simulink model "TestStructure"  (R2023b)
settings: Solver=FixedStepDiscrete  StartTime=0.0  StopTime=inf  FixedStep=SampleTime  RelTol=1e-3
InitFcn:
  | SampleTime = 0.001;
  | ButtonValue=0;
  | load("BusConfig.mat");
undefined symbols (not defined in the file): DiscIntNeverNeededParam
libraries: slrealtimeethercatlib x219, dspfdesign x28, dspstat3 x23, simulink x21, slpidlib x10, dspswit3 x8, commfilt2 x2, dspsigops x1
(part 2 of 8)

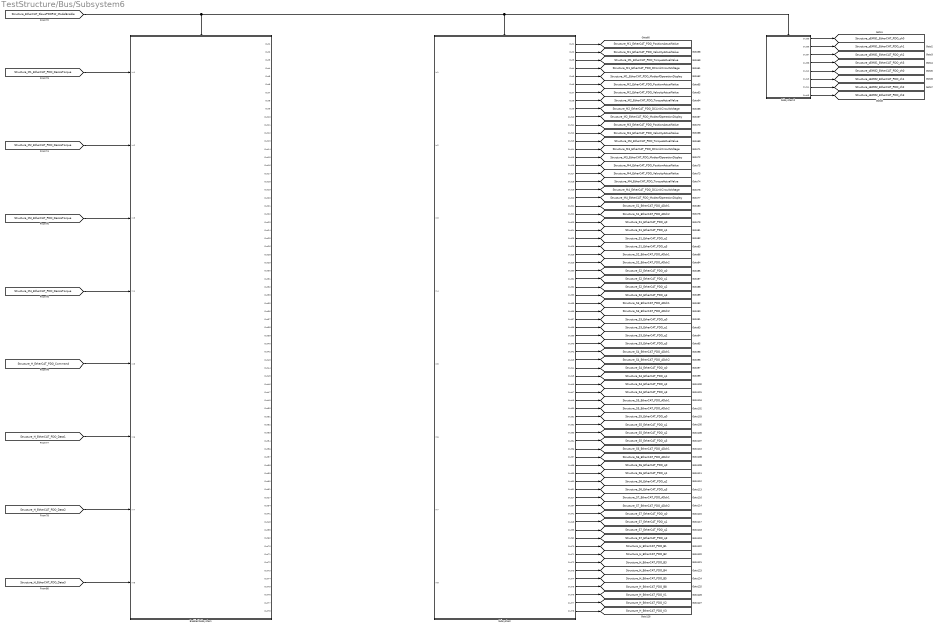
== system TestStructure/Bus/Subsystem6 ==
  Enabled Subsystem : Subsystem  TreatAsAtomicUnit=on
  Subsystem : Subsystem
  Subsystem2 : Subsystem
  tag scope: Structure_H_EtherCAT_PDO_B1=global, Structure_H_EtherCAT_PDO_B2=global, Structure_H_EtherCAT_PDO_B3=global, Structure_H_EtherCAT_PDO_B4=global, Structure_H_EtherCAT_PDO_B5=global, Structure_H_EtherCAT_PDO_B8=global, Structure_H_EtherCAT_PDO_K1=global, Structure_H_EtherCAT_PDO_K2=global, Structure_H_EtherCAT_PDO_K3=global, Structure_M1_EtherCAT_PDO_DCLinkCircuitVoltage=global, Structure_M1_EtherCAT_PDO_ModeofOperationDisplay=global, Structure_M1_EtherCAT_PDO_PositionActualValue=global, Structure_M1_EtherCAT_PDO_TorqueActualValue=global, Structure_M1_EtherCAT_PDO_VelocityActualValue=global, Structure_M2_EtherCAT_PDO_DCLinkCircuitVoltage=global, Structure_M2_EtherCAT_PDO_ModeofOperationDisplay=global, Structure_M2_EtherCAT_PDO_PositionActualValue=global, Structure_M2_EtherCAT_PDO_TorqueActualValue=global, Structure_M2_EtherCAT_PDO_VelocityActualValue=global, Structure_M3_EtherCAT_PDO_DCLinkCircuitVoltage=global, Structure_M3_EtherCAT_PDO_ModeofOperationDisplay=global, Structure_M3_EtherCAT_PDO_PositionActualValue=global, Structure_M3_EtherCAT_PDO_TorqueActualValue=global, Structure_M3_EtherCAT_PDO_VelocityActualValue=global, Structure_M4_EtherCAT_PDO_DCLinkCircuitVoltage=global, Structure_M4_EtherCAT_PDO_ModeofOperationDisplay=global, Structure_M4_EtherCAT_PDO_PositionActualValue=global, Structure_M4_EtherCAT_PDO_TorqueActualValue=global, Structure_M4_EtherCAT_PDO_VelocityActualValue=global, Structure_S1_EtherCAT_PDO_ADch1=global, Structure_S1_EtherCAT_PDO_ADch2=global, Structure_S1_EtherCAT_PDO_q0=global, Structure_S1_EtherCAT_PDO_q1=global, Structure_S1_EtherCAT_PDO_q2=global, Structure_S1_EtherCAT_PDO_q3=global, Structure_S2_EtherCAT_PDO_ADch1=global, Structure_S2_EtherCAT_PDO_ADch2=global, Structure_S2_EtherCAT_PDO_q0=global, Structure_S2_EtherCAT_PDO_q1=global, Structure_S2_EtherCAT_PDO_q2=global, Structure_S2_EtherCAT_PDO_q3=global, Structure_S3_EtherCAT_PDO_ADch1=global, Structure_S3_EtherCAT_PDO_ADch2=global, Structure_S3_EtherCAT_PDO_q0=global, Structure_S3_EtherCAT_PDO_q1=global, Structure_S3_EtherCAT_PDO_q2=global, Structure_S3_EtherCAT_PDO_q3=global, Structure_S4_EtherCAT_PDO_ADch1=global, Structure_S4_EtherCAT_PDO_ADch2=global, Structure_S4_EtherCAT_PDO_q0=global, Structure_S4_EtherCAT_PDO_q1=global, Structure_S4_EtherCAT_PDO_q2=global, Structure_S4_EtherCAT_PDO_q3=global, Structure_S5_EtherCAT_PDO_ADch1=global, Structure_S5_EtherCAT_PDO_ADch2=global, Structure_S5_EtherCAT_PDO_q0=global, Structure_S5_EtherCAT_PDO_q1=global, Structure_S5_EtherCAT_PDO_q2=global, Structure_S5_EtherCAT_PDO_q3=global, Structure_S6_EtherCAT_PDO_ADch1=global, Structure_S6_EtherCAT_PDO_ADch2=global, Structure_S6_EtherCAT_PDO_q0=global, Structure_S6_EtherCAT_PDO_q1=global, Structure_S6_EtherCAT_PDO_q2=global, Structure_S6_EtherCAT_PDO_q3=global, Structure_S7_EtherCAT_PDO_ADch1=global, Structure_S7_EtherCAT_PDO_ADch2=global, Structure_S7_EtherCAT_PDO_q0=global, Structure_S7_EtherCAT_PDO_q1=global, Structure_S7_EtherCAT_PDO_q2=global, Structure_S7_EtherCAT_PDO_q3=global, Structure_sEMG1_EtherCAT_PDO_ch0=global, Structure_sEMG1_EtherCAT_PDO_ch1=global, Structure_sEMG1_EtherCAT_PDO_ch2=global, Structure_sEMG1_EtherCAT_PDO_ch3=global, Structure_sEMG2_EtherCAT_PDO_ch0=global, Structure_sEMG2_EtherCAT_PDO_ch1=global, Structure_sEMG2_EtherCAT_PDO_ch2=global, Structure_sEMG2_EtherCAT_PDO_ch3=global
  wires:
  [Structure_EtherCAT_SlavePDORW_ModelEnable] -> Subsystem2/Enable, Subsystem/Enable, Enabled Subsystem/Enable
  [Structure_M1_EtherCAT_PDO_DesireTorque] -> Enabled Subsystem/1(In1)
  [Structure_M2_EtherCAT_PDO_DesireTorque] -> Enabled Subsystem/2(In2)
  [Structure_M3_EtherCAT_PDO_DesireTorque] -> Enabled Subsystem/3(In3)
  [Structure_M4_EtherCAT_PDO_DesireTorque] -> Enabled Subsystem/4(In4)
  [Structure_H_EtherCAT_PDO_Command] -> Enabled Subsystem/5(In5)
  [Structure_H_EtherCAT_PDO_Data1] -> Enabled Subsystem/6(In6)
  [Structure_H_EtherCAT_PDO_Data2] -> Enabled Subsystem/7(In7)
  [Structure_H_EtherCAT_PDO_Data3] -> Enabled Subsystem/8(In8)
  Subsystem/1(Out1) -> [Structure_M1_EtherCAT_PDO_PositionActualValue]
  Subsystem/2(Out2) -> [Structure_M1_EtherCAT_PDO_VelocityActualValue]
  Subsystem/3(Out3) -> [Structure_M1_EtherCAT_PDO_TorqueActualValue]
  Subsystem/4(Out4) -> [Structure_M1_EtherCAT_PDO_DCLinkCircuitVoltage]
  Subsystem/5(Out5) -> [Structure_M1_EtherCAT_PDO_ModeofOperationDisplay]
  Subsystem/6(Out6) -> [Structure_M2_EtherCAT_PDO_PositionActualValue]
  Subsystem/7(Out7) -> [Structure_M2_EtherCAT_PDO_VelocityActualValue]
  Subsystem/8(Out8) -> [Structure_M2_EtherCAT_PDO_TorqueActualValue]
  Subsystem/9(Out9) -> [Structure_M2_EtherCAT_PDO_DCLinkCircuitVoltage]
  Subsystem/10(Out10) -> [Structure_M2_EtherCAT_PDO_ModeofOperationDisplay]
  Subsystem/11(Out11) -> [Structure_M3_EtherCAT_PDO_PositionActualValue]
  Subsystem/12(Out12) -> [Structure_M3_EtherCAT_PDO_VelocityActualValue]
  Subsystem/13(Out13) -> [Structure_M3_EtherCAT_PDO_TorqueActualValue]
  Subsystem/14(Out14) -> [Structure_M3_EtherCAT_PDO_DCLinkCircuitVoltage]
  Subsystem/15(Out15) -> [Structure_M3_EtherCAT_PDO_ModeofOperationDisplay]
  Subsystem/16(Out16) -> [Structure_M4_EtherCAT_PDO_PositionActualValue]
  Subsystem/17(Out17) -> [Structure_M4_EtherCAT_PDO_VelocityActualValue]
  Subsystem/18(Out18) -> [Structure_M4_EtherCAT_PDO_TorqueActualValue]
  Subsystem/19(Out19) -> [Structure_M4_EtherCAT_PDO_DCLinkCircuitVoltage]
  Subsystem/20(Out20) -> [Structure_M4_EtherCAT_PDO_ModeofOperationDisplay]
  Subsystem/21(Out21) -> [Structure_S1_EtherCAT_PDO_ADch1]
  Subsystem/22(Out22) -> [Structure_S1_EtherCAT_PDO_ADch2]
  Subsystem/23(Out23) -> [Structure_S1_EtherCAT_PDO_q0]
  Subsystem/24(Out24) -> [Structure_S1_EtherCAT_PDO_q1]
  Subsystem/25(Out25) -> [Structure_S1_EtherCAT_PDO_q2]
  Subsystem/26(Out26) -> [Structure_S1_EtherCAT_PDO_q3]
  Subsystem/27(Out28) -> [Structure_S2_EtherCAT_PDO_ADch1]
  Subsystem/28(Out29) -> [Structure_S2_EtherCAT_PDO_ADch2]
  Subsystem/29(Out30) -> [Structure_S2_EtherCAT_PDO_q0]
  Subsystem/30(Out31) -> [Structure_S2_EtherCAT_PDO_q1]
  Subsystem/31(Out32) -> [Structure_S2_EtherCAT_PDO_q2]
  Subsystem/32(Out33) -> [Structure_S2_EtherCAT_PDO_q3]
  Subsystem/33(Out35) -> [Structure_S3_EtherCAT_PDO_ADch1]
  Subsystem/34(Out36) -> [Structure_S3_EtherCAT_PDO_ADch2]
  Subsystem/35(Out37) -> [Structure_S3_EtherCAT_PDO_q0]
  Subsystem/36(Out38) -> [Structure_S3_EtherCAT_PDO_q1]
  Subsystem/37(Out39) -> [Structure_S3_EtherCAT_PDO_q2]
  Subsystem/38(Out40) -> [Structure_S3_EtherCAT_PDO_q3]
  Subsystem/39(Out42) -> [Structure_S4_EtherCAT_PDO_ADch1]
  Subsystem/40(Out43) -> [Structure_S4_EtherCAT_PDO_ADch2]
  Subsystem/41(Out44) -> [Structure_S4_EtherCAT_PDO_q0]
  Subsystem/42(Out45) -> [Structure_S4_EtherCAT_PDO_q1]
  Subsystem/43(Out46) -> [Structure_S4_EtherCAT_PDO_q2]
  Subsystem/44(Out47) -> [Structure_S4_EtherCAT_PDO_q3]
  Subsystem/45(Out49) -> [Structure_S5_EtherCAT_PDO_ADch1]
  Subsystem/46(Out50) -> [Structure_S5_EtherCAT_PDO_ADch2]
  Subsystem/47(Out51) -> [Structure_S5_EtherCAT_PDO_q0]
  Subsystem/48(Out52) -> [Structure_S5_EtherCAT_PDO_q1]
  Subsystem/49(Out53) -> [Structure_S5_EtherCAT_PDO_q2]
  Subsystem/50(Out54) -> [Structure_S5_EtherCAT_PDO_q3]
  Subsystem/51(Out56) -> [Structure_S6_EtherCAT_PDO_ADch1]
  Subsystem/52(Out57) -> [Structure_S6_EtherCAT_PDO_ADch2]
  Subsystem/53(Out58) -> [Structure_S6_EtherCAT_PDO_q0]
  Subsystem/54(Out59) -> [Structure_S6_EtherCAT_PDO_q1]
  Subsystem/55(Out60) -> [Structure_S6_EtherCAT_PDO_q2]
  Subsystem/56(Out61) -> [Structure_S6_EtherCAT_PDO_q3]
  Subsystem/57(Out27) -> [Structure_S7_EtherCAT_PDO_ADch1]
  Subsystem/58(Out34) -> [Structure_S7_EtherCAT_PDO_ADch2]
  Subsystem/59(Out41) -> [Structure_S7_EtherCAT_PDO_q0]
  Subsystem/60(Out48) -> [Structure_S7_EtherCAT_PDO_q1]
  Subsystem/61(Out55) -> [Structure_S7_EtherCAT_PDO_q2]
  Subsystem/62(Out62) -> [Structure_S7_EtherCAT_PDO_q3]
  Subsystem/63(Out70) -> [Structure_H_EtherCAT_PDO_B1]
  Subsystem/64(Out71) -> [Structure_H_EtherCAT_PDO_B2]
  Subsystem/65(Out72) -> [Structure_H_EtherCAT_PDO_B3]
  Subsystem/66(Out73) -> [Structure_H_EtherCAT_PDO_B4]
  Subsystem/67(Out74) -> [Structure_H_EtherCAT_PDO_B5]
  Subsystem/68(Out75) -> [Structure_H_EtherCAT_PDO_B8]
  Subsystem/69(Out76) -> [Structure_H_EtherCAT_PDO_K1]
  Subsystem/70(Out77) -> [Structure_H_EtherCAT_PDO_K2]
  Subsystem/71(Out78) -> [Structure_H_EtherCAT_PDO_K3]
  Subsystem2/1(Out35) -> [Structure_sEMG1_EtherCAT_PDO_ch0]
  Subsystem2/2(Out36) -> [Structure_sEMG1_EtherCAT_PDO_ch1]
  Subsystem2/3(Out37) -> [Structure_sEMG1_EtherCAT_PDO_ch2]
  Subsystem2/4(Out38) -> [Structure_sEMG1_EtherCAT_PDO_ch3]
  Subsystem2/5(Out42) -> [Structure_sEMG2_EtherCAT_PDO_ch0]
  Subsystem2/6(Out43) -> [Structure_sEMG2_EtherCAT_PDO_ch1]
  Subsystem2/7(Out44) -> [Structure_sEMG2_EtherCAT_PDO_ch2]
  Subsystem2/8(Out45) -> [Structure_sEMG2_EtherCAT_PDO_ch3]

== system TestStructure/Bus/Subsystem7 ==
  Enabled Subsystem : Subsystem  Commented=on  TreatAsAtomicUnit=on
  Enabled Subsystem1 : Subsystem  Commented=on  TreatAsAtomicUnit=on
  Enabled Subsystem2 : Subsystem  Commented=on  TreatAsAtomicUnit=on
  Enabled Subsystem3 : Subsystem  Commented=on  TreatAsAtomicUnit=on
  Enabled Subsystem4 : Subsystem  Commented=on  TreatAsAtomicUnit=on
  Enabled Subsystem5 : Subsystem  Commented=on  TreatAsAtomicUnit=on
  Enabled Subsystem6 : Subsystem  Commented=on  TreatAsAtomicUnit=on
  Enabled Subsystem7 : Subsystem  Commented=on  TreatAsAtomicUnit=on
  tag scope: Structure_M4_EtherCAT_GetDeviceState_State=global, Structure_M4_EtherCAT_Init_PDO_PositionActualValue=global, Structure_M4_EtherCAT_PDO_StatusWord=global, Structure_M4_EtherCAT_SDO_6060_Error=global, Structure_M4_EtherCAT_SDO_6060_Status=global, Structure_M4_EtherCAT_SDO_6075_Data=global, Structure_M4_EtherCAT_SDO_6075_Error=global, Structure_M4_EtherCAT_SDO_6075_Status=global, Structure_M4_EtherCAT_SDO_6080_Error=global, Structure_M4_EtherCAT_SDO_6080_Status=global, Structure_M4_EtherCAT_SetDeviceState1_Error=global, Structure_M4_EtherCAT_SetDeviceState1_PrevState=global, Structure_M4_EtherCAT_SetDeviceState_Error=global, Structure_M4_EtherCAT_SetDeviceState_PrevState=global
  wires:
  [Structure_M4_EtherCAT_SetDeviceState_ModelEnable] -> Enabled Subsystem/Enable
  [Structure_M4_EtherCAT_SDO_6075_ModelEnable] -> Enabled Subsystem1/Enable
  [Structure_M4_EtherCAT_SDO_6080_ModelEnable] -> Enabled Subsystem2/Enable
  [Structure_M4_EtherCAT_SDO_6060_ModelEnable] -> Enabled Subsystem3/Enable
  [Structure_M4_EtherCAT_SetDeviceState1_ModelEnable] -> Enabled Subsystem4/Enable
  [Structure_M4_EtherCAT_InitReadPos_ModelEnable] -> Enabled Subsystem7/Enable
  [Structure_M4_EtherCAT_PDO_6040_ModelEnable] -> Enabled Subsystem6/Enable
  [Structure_M4_EtherCAT_GetDeviceState_ModelEnable] -> Enabled Subsystem5/Enable
  [Structure_M4_EtherCAT_SetDeviceState_NewState] -> Enabled Subsystem/1(In1)
  [Structure_M4_EtherCAT_SetDeviceState_Enable] -> Enabled Subsystem/2(In2)
  Enabled Subsystem/1(Out1) -> [Structure_M4_EtherCAT_SetDeviceState_PrevState]
  Enabled Subsystem/2(Out2) -> [Structure_M4_EtherCAT_SetDeviceState_Error]
  [Structure_M4_EtherCAT_SDO_6075_Enable] -> Enabled Subsystem1/1(In3)
  Enabled Subsystem1/1(Out3) -> [Structure_M4_EtherCAT_SDO_6075_Data]
  Enabled Subsystem1/2(Out4) -> [Structure_M4_EtherCAT_SDO_6075_Status]
  Enabled Subsystem1/3(Out5) -> [Structure_M4_EtherCAT_SDO_6075_Error]
  [Structure_M4_EtherCAT_SDO_6080_Enable] -> Enabled Subsystem2/2(In5)
  [Structure_M4_EtherCAT_SDO_6080_Data] -> Enabled Subsystem2/1(In4)
  Enabled Subsystem2/2(Out7) -> [Structure_M4_EtherCAT_SDO_6080_Error]
  Enabled Subsystem2/1(Out6) -> [Structure_M4_EtherCAT_SDO_6080_Status]
  [Structure_M4_EtherCAT_SDO_6060_Data] -> Enabled Subsystem3/1(In6)
  [Structure_M4_EtherCAT_SDO_6060_Enable] -> Enabled Subsystem3/2(In7)
  Enabled Subsystem3/1(Out8) -> [Structure_M4_EtherCAT_SDO_6060_Status]
  Enabled Subsystem3/2(Out9) -> [Structure_M4_EtherCAT_SDO_6060_Error]
  [Structure_M4_EtherCAT_SetDeviceState1_NewState] -> Enabled Subsystem4/1(In8)
  [Structure_M4_EtherCAT_SetDeviceState1_Enable] -> Enabled Subsystem4/2(In9)
  Enabled Subsystem4/1(Out10) -> [Structure_M4_EtherCAT_SetDeviceState1_PrevState]
  Enabled Subsystem4/2(Out11) -> [Structure_M4_EtherCAT_SetDeviceState1_Error]
  Enabled Subsystem5/1(Out12) -> [Structure_M4_EtherCAT_GetDeviceState_State]
  [Structure_M4_EtherCAT_PDO_ControlWord] -> Enabled Subsystem6/1(In10)
  Enabled Subsystem6/1(Out13) -> [Structure_M4_EtherCAT_PDO_StatusWord]
  Enabled Subsystem7/1(Out1) -> [Structure_M4_EtherCAT_Init_PDO_PositionActualValue]

== system TestStructure/InterForceControlTask/AO ==
  q : Inport
  sEMGMuxIn : Inport  Port=2
  PhaseBias : Inport  Port=3
  Whichfoot : Inport  Port=4
  ColdStartEventClock : DigitalClock  SampleTime=0.001
  ColdStartEventGate : MATLAB Function  TreatAsAtomicUnit=on
  Constant : Constant
  Constant1 : Constant
  Demux : Demux  Outputs=3
  Filter : Subsystem
  Gain : Gain  Gain=0.01
  MATLAB Function : MATLAB Function  TreatAsAtomicUnit=on
  Memory : Memory
  PhaseCorrection : Subsystem
      settings: PortSchema="{\"entries\":[{\"content\":{\"sides\":[{\"content\":{\"connectorIds\":[\"In1\"]},\"type\":\"ConnectorPlacement.EquallySpacedRectSide\",\"uuid\":\"a940d053-290e-486f-ae2d-d4bfa32c46e0\"},{\"content\":{\"connectorIds\":[\"Out1\",\"Out2\"],\"side\":\"RIGHT\"},\"type\":\"ConnectorPlacement.EquallySpacedRectSide\",\"uuid\":\"a83f9ff7-c6c8-4eeb-9804-d4a4971b2c0c\"},{\"content\":{\"side\":\"TOP\"},\"type\":\"ConnectorPlacement.EquallySpacedRectSide\",\"uuid\":\"31fb4f87-600a-4f18-9d17-ff98d57e3413\"},{\"content\":{\"connectorIds\":[\"In2\"],\"side\":\"BOTTOM\"},\"type\":\"ConnectorPlacement.EquallySpacedRectSide\",\"uuid\":\"7c261045-8ba1-4ca6-a6a7-b959d0e37f01\"}]},\"type\":\"ConnectorPlacement.EquallySpacedConnector\",\"uuid\":\"19432f00-0669-4bb6-9210-56124374c33b\"}],\"packageUris\":[\"http://schema.mathworks.com/mf0/Connector/R2020b\"],\"version\":\"1.0\"}"
  Select : Subsystem
  Subsystem1 : Subsystem
  Switch : Switch  Criteria=u2 > Threshold  SaturateOnIntegerOverflow=off  InputSameDT=off
  TBaseDefault : Constant  Value=2.2
  FeetLoad : Outport
  x : Outport  Port=2
  Omega : Outport  Port=3
  Phi : Outport  Port=4
  Phase0Event : Outport  Port=5
  wires:
  Memory/1 -> MATLAB Function/1(phi)
  Select/3(PhaseEn) -> Subsystem1/Enable
  Constant1/1 -> Select/1(P)
  PhaseCorrection/1(Omega) -> Omega/1
  Gain/1 -> Select/3(q), Subsystem1/1(q)
  Select/1(Phi_Out) -> Phi/1
  MATLAB Function/1(y) -> Select/2(Phi)
  PhaseCorrection/2(Phi_Corrected) -> Memory/1
  PhaseBias/1 -> MATLAB Function/2(deltaphi)
  Filter/1(Out) -> Gain/1
  Subsystem1/2(Peak) -> PhaseCorrection/1(Peaks)
  sEMGMuxIn/1 -> Subsystem1/2(sEMGMuxIn)
  Whichfoot/1 -> Subsystem1/3(Whichfoot)
  Subsystem1/3(FeetLoad) -> FeetLoad/1
  q/1 -> Demux/1
  Demux/2 -> Switch/2  "which"
  Demux/1 -> Switch/1  "left"
  Demux/3 -> Switch/3  "right"
  Switch/1 -> Filter/1(In)
  TBaseDefault/1 -> PhaseCorrection/2(T_base_default), ColdStartEventGate/3(T_base_default)
  Select/2(Phase0Event) -> Phase0Event/1, ColdStartEventGate/1(event_in)
  ColdStartEventClock/1 -> ColdStartEventGate/2(t_now)
  ColdStartEventGate/1(event_out) -> ?

== system TestStructure/InterForceControlTask/AO1 ==
  q : Inport
  PhaseBias : Inport  Port=2
  Bias : Bias  Bias=-30  SaturateOnIntegerOverflow=off
  Constant : Constant
  Constant1 : Constant
  Filter : Subsystem
  Gain : Gain  Gain=0.01
  MATLAB Function : MATLAB Function  TreatAsAtomicUnit=on
  Memory : Memory
  PhaseCorrection : Subsystem
  Select : Subsystem
  Subsystem : Subsystem  Commented=on
  Subsystem1 : Subsystem
  x : Outport
  Omega : Outport  Port=2
  Phi : Outport  Port=3
  Phase0Event : Outport  Port=4
  wires:
  Memory/1 -> MATLAB Function/1(phi)
  Subsystem1/2(Peak) -> PhaseCorrection/1(Peaks)
  Select/3(PhaseEn) -> Subsystem1/Enable
  Constant1/1 -> Select/1(P)
  PhaseCorrection/1(Omega) -> Omega/1
  Gain/1 -> Subsystem1/1(q), Select/3(q)
  Select/2(Phase0Event) -> Phase0Event/1
  Select/1(Phi_Out) -> Phi/1
  MATLAB Function/1(y) -> Select/2(Phi)
  PhaseCorrection/2(Phi_Corrected) -> Memory/1
  PhaseBias/1 -> MATLAB Function/2(deltaphi)
  Bias/1 -> ?
  Filter/1(Out) -> Gain/1, Bias/1
  q/1 -> Filter/1(In)

== system TestStructure/InterForceControlTask/AO2 ==
  q : Inport
  PhaseBias : Inport  Port=2
  Bias : Bias  Bias=-30  SaturateOnIntegerOverflow=off
  Filter : Subsystem
  Gain : Gain  Gain=0.01
  MATLAB Function : MATLAB Function  TreatAsAtomicUnit=on
  PhaseCorrection : Subsystem
      settings: PortSchema="{\"entries\":[{\"content\":{\"sides\":[{\"content\":{\"connectorIds\":[\"In1\"]},\"type\":\"ConnectorPlacement.EquallySpacedRectSide\",\"uuid\":\"29c766a6-008c-4672-8933-7f2b92d9002e\"},{\"content\":{\"connectorIds\":[\"Out1\"],\"side\":\"RIGHT\"},\"type\":\"ConnectorPlacement.EquallySpacedRectSide\",\"uuid\":\"ebf4015b-900d-44c2-b090-12eb3718c736\"},{\"content\":{\"connectorIds\":[\"In2\",\"In3\",\"In4\"],\"side\":\"TOP\"},\"type\":\"ConnectorPlacement.EquallySpacedRectSide\",\"uuid\":\"76801015-3401-4c32-9066-c2a5e8571b2e\"},{\"content\":{\"side\":\"BOTTOM\"},\"type\":\"ConnectorPlacement.EquallySpacedRectSide\",\"uuid\":\"4a70095e-69af-4392-aa02-795a2e72b843\"}]},\"type\":\"ConnectorPlacement.EquallySpacedConnector\",\"uuid\":\"005c6ef6-da38-46d8-8867-20bf9861f3d8\"}],\"packageUris\":[\"http://schema.mathworks.com/mf0/Connector/R2020b\"],\"version\":\"1.0\"}"
  Select : Subsystem
  Subsystem : Subsystem
  Subsystem1 : Subsystem
  x : Outport
  Omega : Outport  Port=2
  Phi : Outport  Port=3
  Phase0Event : Outport  Port=4
  wires:
  Select/2(Phase0Event) -> Phase0Event/1
  Select/1(Phi_Out) -> Phi/1
  MATLAB Function/1(y) -> Select/2(Phi)
  Subsystem/4(P) -> Select/1(P)
  PhaseCorrection/1(Phi_Corrected) -> MATLAB Function/1(phi)
  Subsystem/3(Phi) -> PhaseCorrection/2(Phi_GP)
  Subsystem/2(Omega) -> PhaseCorrection/3(Omega), Omega/1
  PhaseBias/1 -> MATLAB Function/2(deltaphi)
  Subsystem1/1(f) -> Subsystem/2(f)
  Bias/1 -> ?
  Gain/1 -> Subsystem1/1(q), Select/3(q), Subsystem/1(q)
  Filter/1(Out) -> Gain/1, Bias/1
  Subsystem1/2(Peak) -> PhaseCorrection/1(Peaks)
  q/1 -> Filter/1(In)
  Subsystem/1(x) -> x/1

== system TestStructure/InterForceControlTask/AO3 ==
  q : Inport
  PhaseBias : Inport  Port=2
  Bias : Bias  Bias=-30  SaturateOnIntegerOverflow=off
  Constant : Constant
  Constant1 : Constant
  Filter : Subsystem
  Gain : Gain  Gain=0.01
  MATLAB Function : MATLAB Function  TreatAsAtomicUnit=on
  PhaseCorrection : Subsystem
  Select : Subsystem
  Subsystem : Subsystem  Commented=on
  Subsystem1 : Subsystem
  x : Outport
  Omega : Outport  Port=2
  Phi : Outport  Port=3
  Phase0Event : Outport  Port=4
  wires:
  Constant1/1 -> Select/1(P)
  PhaseCorrection/1(Omega) -> Omega/1
  Constant/1 -> Select/3(q)
  Select/2(Phase0Event) -> Phase0Event/1
  Select/1(Phi_Out) -> Phi/1
  MATLAB Function/1(y) -> Select/2(Phi)
  PhaseCorrection/2(Phi_Corrected) -> MATLAB Function/1(phi)
  PhaseBias/1 -> MATLAB Function/2(deltaphi)
  Bias/1 -> ?
  Gain/1 -> Subsystem1/1(q)
  Filter/1(Out) -> Gain/1, Bias/1
  Subsystem1/2(Peak) -> PhaseCorrection/1(Peaks)
  q/1 -> Filter/1(In)

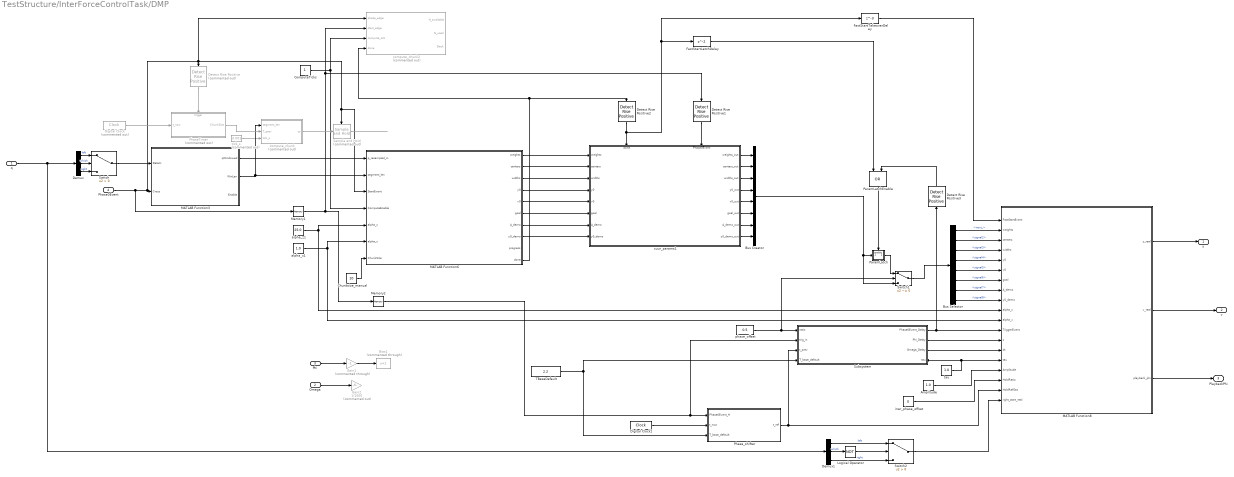
== system TestStructure/InterForceControlTask/DMP ==
  q : Inport
  Omega : Inport  Port=2
  Phi : Inport  Port=3
  Phase0Event : Inport  Port=4
  Amplitude : Constant  Value=1.0
  Bias1 : Bias  Commented=through  Bias=1  SaturateOnIntegerOverflow=off
  Bus Creator : BusCreator  Inputs=8
  Bus Selector : BusSelector  OutputSignals=next_,signal2,signal3,signal4,signal5,signal6,signal7,signal8
  Chunksize_manual : Constant  Value=10
  ComputeTicks : Constant
  Demux : Demux  Outputs=3
  Demux1 : Demux  Outputs=3
  Detect Rise Positive : simulink/Logic and Bit Operations/Detect Rise Positive  Commented=on  vinit=0  OutDataTypeStr=boolean
  Detect Rise Positive1 : simulink/Logic and Bit Operations/Detect Rise Positive  vinit=0  OutDataTypeStr=boolean
  Detect Rise Positive2 : simulink/Logic and Bit Operations/Detect Rise Positive  vinit=0  OutDataTypeStr=boolean
  Detect Rise Positive3 : simulink/Logic and Bit Operations/Detect Rise Positive  vinit=0  OutDataTypeStr=boolean
  Digital Clock : DigitalClock  Commented=on  SampleTime=0.001
  Digital Clock1 : DigitalClock  SampleTime=0.001
  FastStartLatchDelay : Delay  InitialCondition=0
  FastStartTakeoverDelay : Delay  DelayLength=3  InitialCondition=0
  Gain1 : Gain  Commented=through  Gain=-1
  Gain2 : Gain  Commented=on  Gain=1/1000
  Logical Operator : Logic  Operator=NOT  AllPortsSameDT=off  OutDataTypeStr=boolean
  MATLAB Function3 : MATLAB Function  TreatAsAtomicUnit=on
  MATLAB Function6 : MATLAB Function  TreatAsAtomicUnit=on
  MATLAB Function8 : MATLAB Function  TreatAsAtomicUnit=on
  Memory1 : Memory
  Memory2 : Memory
  ParamLatch : Subsystem  TreatAsAtomicUnit=on
  ParamLatchEnable : Logic  Operator=OR  AllPortsSameDT=off  OutDataTypeStr=boolean
  PhaseTimer : Subsystem  Commented=on  TreatAsAtomicUnit=on
  Phase_shifter : MATLAB Function  TreatAsAtomicUnit=on
  Sample and Hold : dspsigops/Sample and Hold  Commented=on  trig=Rising edge  initCond=0  latchinput=off
  Subsystem : Subsystem
      settings: PortSchema="{\"entries\":[{\"content\":{\"sides\":[{\"content\":{\"connectorIds\":[\"In1\",\"In2\",\"In3\",\"In4\"]},\"type\":\"ConnectorPlacement.EquallySpacedRectSide\",\"uuid\":\"1070cfcb-3ec5-4141-8951-8c3ef1706a2a\"},{\"content\":{\"connectorIds\":[\"Out1\",\"Out2\",\"Out3\",\"In5\"],\"side\":\"RIGHT\"},\"type\":\"ConnectorPlacement.EquallySpacedRectSide\",\"uuid\":\"bed4e625-42d0-4ea4-b6d1-bbd729333a1c\"},{\"content\":{\"side\":\"TOP\"},\"type\":\"ConnectorPlacement.EquallySpacedRectSide\",\"uuid\":\"c279c2b1-2727-4963-bce9-c67f4ee7a970\"}]},\"type\":\"ConnectorPlacement.EquallySpacedConnector\",\"uuid\":\"94e6fa59-a73d-4cda-bb27-ca572fd247c8\"}],\"packageUris\":[\"http://schema.mathworks.com/mf0/Connector/R2020b\"],\"version\":\"1.0\"}"
  Switch : Switch  Criteria=u2 > Threshold  SaturateOnIntegerOverflow=off  InputSameDT=off
  Switch1 : Switch  Criteria=u2 ~= 0  SaturateOnIntegerOverflow=off  InputSameDT=off
  Switch2 : Switch  Criteria=u2 > Threshold  SaturateOnIntegerOverflow=off  InputSameDT=off
  TBaseDefault : Constant  Value=2.2
  alpha_x1 : Constant  Value=1.0
  alpha_z1 : Constant  Value=25.0
  compute_chunk : MATLAB Function  Commented=on  TreatAsAtomicUnit=on
  compute_chunk2 : MATLAB Function  Commented=on  TreatAsAtomicUnit=on
  cuur_params1 : Subsystem  TreatAsAtomicUnit=on
      settings: PortSchema="{\"entries\":[{\"content\":{\"sides\":[{\"content\":{\"connectorIds\":[\"In1\",\"In2\",\"In3\",\"In4\",\"In5\",\"In6\",\"In7\",\"In8\"]},\"type\":\"ConnectorPlacement.EquallySpacedRectSide\",\"uuid\":\"3d372f5a-e7b4-49e3-b2c9-9176d5cbfa33\"},{\"content\":{\"connectorIds\":[\"Out1\",\"Out2\",\"Out3\",\"Out4\",\"Out5\",\"Out6\",\"Out7\",\"Out8\"],\"side\":\"RIGHT\"},\"type\":\"ConnectorPlacement.EquallySpacedRectSide\",\"uuid\":\"ee9298d3-2ae2-4770-892a-2c75b17955ec\"},{\"content\":{\"connectorIds\":[\"In9\",\"In10\"],\"side\":\"TOP\"},\"type\":\"ConnectorPlacement.EquallySpacedRectSide\",\"uuid\":\"d0638e77-81ba-40cc-8800-354c93838fef\"}]},\"type\":\"ConnectorPlacement.EquallySpacedConnector\",\"uuid\":\"50317f07-3edb-4206-bc08-c56b750c0251\"}],\"packageUris\":[\"http://schema.mathworks.com/mf0/Connector/R2020b\"],\"version\":\"1.0\"}"
  iner_phase_offset : Constant  Value=0
  phase_offset : Constant  Value=0.5
  tau : Constant  Value=1.0
  tick_s : Constant  Commented=on  Value=0.001
  y : Outport
  v : Outport  Port=2
  PlaybackPhi : Outport  Port=3
  wires:
  MATLAB Function8/2(v_real) -> v/1
  Subsystem/2(Phi_Delay) -> MATLAB Function8/13(s)
  Subsystem/1(Phase0Event_Delay) -> MATLAB Function8/12(TriggerEvent), Detect Rise Positive3/1
  Subsystem/3(Omega_Delay) -> MATLAB Function8/14(dt)
  Bus Selector/8 -> MATLAB Function8/9(y0_demo)  "<signal8>"
  Bus Selector/7 -> MATLAB Function8/8(A_demo)  "<signal7>"
  Bus Selector/6 -> MATLAB Function8/7(goal)  "<signal6>"
  Bus Selector/5 -> MATLAB Function8/6(v0)  "<signal5>"
  Bus Selector/4 -> MATLAB Function8/5(y0)  "<signal4>"
  Bus Selector/3 -> MATLAB Function8/4(widths)  "<signal3>"
  Bus Selector/2 -> MATLAB Function8/3(centers)  "<signal2>"
  Bus Selector/1 -> MATLAB Function8/2(weights)  "<next_>"
  Switch1/1 -> Bus Selector/1
  ParamLatch/1(Out1) -> Switch1/1
  phase_offset/1 -> Switch1/2, Subsystem/1(ratio)
  Detect Rise Positive3/1 -> ParamLatchEnable/2
  Bus Creator/1 -> Switch1/3, ParamLatch/1(In1)
  MATLAB Function8/1(y_real) -> y/1
  cuur_params1/8(y0_demo_out) -> Bus Creator/8
  cuur_params1/7(A_demo_out) -> Bus Creator/7
  cuur_params1/6(goal_out) -> Bus Creator/6
  cuur_params1/5(v0_out) -> Bus Creator/5
  cuur_params1/4(y0_out) -> Bus Creator/4
  cuur_params1/3(widths_out) -> Bus Creator/3
  cuur_params1/2(centers_out) -> Bus Creator/2
  cuur_params1/1(weights_out) -> Bus Creator/1
  iner_phase_offset/1 -> MATLAB Function8/17(HoldRatio)
  Phase_shifter/1(t_ref) -> MATLAB Function8/18(HoldRefSec), Subsystem/3(t_prev)
  Digital Clock1/1 -> Phase_shifter/2(t_now)
  Chunksize_manual/1 -> MATLAB Function6/7(ChunkSize)
  ComputeTicks/1 -> MATLAB Function6/4(ComputeEnable), compute_chunk2/3(compute_tick)
  q/1 -> Demux1/1, Demux/1
  MATLAB Function6/2(centers) -> cuur_params1/2(centers)
  Gain1/1 -> Bias1/1
  MATLAB Function6/6(goal) -> cuur_params1/6(goal)
  Phase0Event/1 -> Memory1/1, MATLAB Function3/2(Cross), Detect Rise Positive/1, MATLAB Function6/3(StartEvent), Sample and Hold/Trigger, compute_chunk2/1(phase_edge)
  MATLAB Function3/1(qWindowed) -> MATLAB Function6/1(p_resampled_in)
  alpha_x1/1 -> MATLAB Function6/6(alpha_x), MATLAB Function8/11(alpha_x)
  Digital Clock/1 -> PhaseTimer/1(t_now)
  tick_s/1 -> compute_chunk/3(tick_s)
  alpha_z1/1 -> MATLAB Function6/5(alpha_z), MATLAB Function8/10(alpha_z)
  Omega/1 -> Gain2/1
  MATLAB Function6/7(A_demo) -> cuur_params1/7(A_demo)
  MATLAB Function6/5(v0) -> cuur_params1/5(v0)
  MATLAB Function3/2(WinLen) -> MATLAB Function6/2(segment_len), compute_chunk/1(segment_len)
  Memory1/1 -> Memory2/1, compute_chunk2/2(start_edge), Detect Rise Positive1/1
  tau/1 -> MATLAB Function8/15(tau), Subsystem/5(tau)
  Amplitude/1 -> MATLAB Function8/16(Amplitude)
  Sample and Hold/1 -> ?
  Detect Rise Positive/1 -> PhaseTimer/Trigger
  MATLAB Function6/8(y0_demo) -> cuur_params1/8(y0_demo)
  Phi/1 -> Gain1/1
  Detect Rise Positive2/1 -> FastStartLatchDelay/1, FastStartTakeoverDelay/1, cuur_params1/9(done)
  MATLAB Function6/4(y0) -> cuur_params1/4(y0)
  MATLAB Function6/1(weights) -> cuur_params1/1(weights)
  MATLAB Function6/10(done) -> Detect Rise Positive2/1, compute_chunk2/4(done)
  Detect Rise Positive1/1 -> cuur_params1/10(Phase0Event)
  compute_chunk/1(cs) -> Sample and Hold/1
  PhaseTimer/1(ChunkSize) -> compute_chunk/2(T_prev)
  Memory2/1 -> Phase_shifter/1(Phase0Event_H), Subsystem/2(trig_in)
  MATLAB Function6/3(widths) -> cuur_params1/3(widths)
  Switch2/1 -> MATLAB Function8/19(right_start_real)
  MATLAB Function8/3(playback_phi) -> PlaybackPhi/1
  TBaseDefault/1 -> Phase_shifter/3(T_base_default), Subsystem/4(T_base_default)
  FastStartLatchDelay/1 -> ParamLatchEnable/1
  ParamLatchEnable/1 -> ParamLatch/Enable
  FastStartTakeoverDelay/1 -> MATLAB Function8/1(FastStartEvent)
  Demux/3 -> Switch/3  "right"
  Demux/2 -> Switch/2  "which"
  Demux/1 -> Switch/1  "left"
  Switch/1 -> MATLAB Function3/1(DataIn)
  Demux1/3 -> Switch2/3  "right"
  Demux1/2 -> Logical Operator/1  "which"
  Demux1/1 -> Switch2/1  "left"
  Logical Operator/1 -> Switch2/2

== system TestStructure/InterForceControlTask/FootSwitch ==
  <LeftHipMotorActuralPosition> : Inport
  <LeftHipMotorActuralVelocity> : Inport  Port=2
  <RightHipMotorActuralPosition> : Inport  Port=3
  <RightHipMotorActuralVelocity> : Inport  Port=4
  <FootSelect> : Inport  Port=5
  Mux : Mux  Inputs=3
  Switch1 : Switch  Criteria=u2 > Threshold  SaturateOnIntegerOverflow=off  InputSameDT=off
  Switch2 : Switch  Criteria=u2 > Threshold  SaturateOnIntegerOverflow=off  InputSameDT=off
  ActuralPosition : Outport
  ActuralVelocity : Outport  Port=2
  q : Outport  Port=3
  wires:
  <LeftHipMotorActuralPosition>/1 -> Mux/1, Switch1/3
  <LeftHipMotorActuralVelocity>/1 -> Switch2/3
  <RightHipMotorActuralPosition>/1 -> Switch1/1, Mux/3
  <RightHipMotorActuralVelocity>/1 -> Switch2/1
  <FootSelect>/1 -> Mux/2, Switch2/2, Switch1/2
  Mux/1 -> q/1
  Switch1/1 -> ActuralPosition/1
  Switch2/1 -> ActuralVelocity/1

== system TestStructure/InterForceControlTask/TorqueController ==
  q_meas : Inport
  dq_meas : Inport  Port=2
  q_ref : Inport  Port=3
  dq_ref : Inport  Port=4
  Abs : Abs  SaturateOnIntegerOverflow=off
  Activity gate : Merge
  Activity_Enable : Constant
  Clock : Clock
  Filter1 : Subsystem
  Gain : Gain  Gain=0.01
  Gain3 : Gain  Gain=0.4
  If : If  NumInputs=2  IfExpression=(u1 >= u2)
  If Action Subsystem1 : Subsystem  TreatAsAtomicUnit=on
  If Action Subsystem_activity_on : Subsystem  TreatAsAtomicUnit=on
  MATLAB Function1 : MATLAB Function  TreatAsAtomicUnit=on
  MATLAB Function2 : MATLAB Function  TreatAsAtomicUnit=on
  MATLAB Function3 : MATLAB Function  TreatAsAtomicUnit=on
  MO_ActivityMovent : Sum
  MO_ActivtyThreadhold : Constant  Value=0.1
  MO_AutoDisable? : ManualSwitch  CurrentSetting=0
  MO_Kd : Gain  Gain=0.002
  MO_Kp : Gain  Gain=0.15
  Moving Average1 : dspstat3/Moving Average  Method=Sliding window  ForgettingFactorPort=off  SpecifyWindowLength=on  WindowLength=2000  OverlapLength=1999  AllowArbitraryInputLength=off  ForgettingFactor=0.9  SimulateUsing=Code generation
  Subsystem2 : Subsystem
  Sum_e : Sum  Inputs=|++
  Sum_e_dq : Sum  Inputs=|-+
  Sum_e_q : Sum  Inputs=|-+
  TorqueManager : Subsystem
  tau_e : Outport
  wires:
  dq_meas/1 -> Sum_e_dq/1
  q_ref/1 -> Filter1/1(In), Sum_e_q/2
  dq_ref/1 -> Sum_e_dq/2
  Sum_e_q/1 -> MO_Kp/1
  Sum_e_dq/1 -> MO_Kd/1
  MO_Kp/1 -> Sum_e/1
  MO_Kd/1 -> Sum_e/2
  Filter1/1(Out) -> Gain/1
  q_meas/1 -> Sum_e_q/1
  Sum_e/1 -> TorqueManager/3(target_torque)
  Subsystem2/1(Peak) -> TorqueManager/2(valid_peak), MATLAB Function2/1(valid_peak), MATLAB Function1/1(raw_peak)  "MO_DMPPhase0Event"
  Clock/1 -> MATLAB Function1/2(t)
  Gain/1 -> MATLAB Function3/1(u), Subsystem2/1(q)
  Gain3/1 -> MO_ActivityMovent/1
  Abs/1 -> Gain3/1, Moving Average1/1
  Moving Average1/1 -> MO_ActivityMovent/2
  If Action Subsystem1/1(activity_gain) -> Activity gate/1  "1"
  MATLAB Function3/1(y) -> Abs/1
  MO_ActivityMovent/1 -> If/1
  If/1 -> If Action Subsystem1/Action
  MO_ActivtyThreadhold/1 -> If/2
  If/2 -> If Action Subsystem_activity_on/Action
  TorqueManager/1(actual_torque) -> tau_e/1
  If Action Subsystem_activity_on/1(activity_gain) -> Activity gate/2  "0"
  Activity gate/1 -> MO_AutoDisable?/1
  TorqueManager/2(current_gain) -> ?  "MO_currentgain"
  MATLAB Function2/1(total_steps) -> ?  "MO_DMPStepCunter"
  Activity_Enable/1 -> MO_AutoDisable?/2
  MO_AutoDisable?/1 -> TorqueManager/1(activity_enable)

== system TestStructure/InterForceControlTask/TorqueController2 ==
  dq_meas : Inport
  q_meas : Inport  Port=2
  q_ref : Inport  Port=3
  dq_ref : Inport  Port=4
  Clock : Clock
  Filter : Subsystem
  Gain : Gain  Gain=0.01
  Gain_Kd : Gain  Gain=0.005
  Gain_Kp : Gain  Gain=0.3
  MATLAB Function : MATLAB Function  TreatAsAtomicUnit=on
  MATLAB Function1 : MATLAB Function  TreatAsAtomicUnit=on
  MATLAB Function2 : MATLAB Function  TreatAsAtomicUnit=on
  Sum_e : Sum  Inputs=|++
  Sum_e_dq : Sum  Inputs=|-+
  Sum_e_q : Sum  Inputs=|-+
  ZeroCrossFinder_Right : Subsystem
  tau_e : Outport
  wires:
  Clock/1 -> MATLAB Function1/2(t), MATLAB Function/3(t)
  MATLAB Function1/1(valid_peak) -> MATLAB Function/1(valid_peak), MATLAB Function2/1(valid_peak)  "valid_peak_right"
  ZeroCrossFinder_Right/1(peak_right) -> MATLAB Function1/1(raw_peak)  "peak_right"
  MATLAB Function/1(actual_torque) -> tau_e/1
  Gain/1 -> ZeroCrossFinder_Right/1(U)
  q_meas/1 -> Sum_e_q/1
  Filter/1(Out) -> Gain/1
  Sum_e/1 -> MATLAB Function/2(target_torque)
  Gain_Kd/1 -> Sum_e/2
  Gain_Kp/1 -> Sum_e/1
  Sum_e_dq/1 -> Gain_Kd/1
  Sum_e_q/1 -> Gain_Kp/1
  dq_ref/1 -> Sum_e_dq/2
  q_ref/1 -> Sum_e_q/2, Filter/1(q)
  dq_meas/1 -> Sum_e_dq/1

== system TestStructure/InterForceControlTask/Torque_Guard ==
  FeetLoad : Inport
  WhichFoot : Inport  Port=2
  tau_e : Inport  Port=3
  <LeftHipMotorActuralPosition> : Inport  Port=4
  <RightHipMotorActuralPosition> : Inport  Port=5
  "?AllTimeDefault" : ManualSwitch
  ContactRelay : Relay  OnSwitchValue=2.0  OffSwitchValue=1.25
  ContactRelay1 : Relay  OnSwitchValue=2.0  OffSwitchValue=1.25
  Demux : Demux  Outputs=2
  Demux1 : Demux  Outputs=2
  LeftLowPass : DiscreteTransferFcn  Numerator=0.05  Denominator=[1 -0.95]  SampleTime=0.001
  LeftLowPass1 : DiscreteTransferFcn  Numerator=0.05  Denominator=[1 -0.95]  SampleTime=0.001
  LimitProtect : Subsystem
      settings: PortSchema="{\"entries\":[{\"content\":{\"sides\":[{\"content\":{\"connectorIds\":[\"In1\",\"In2\",\"In3\"]},\"type\":\"ConnectorPlacement.EquallySpacedRectSide\",\"uuid\":\"37de08c4-f478-48e2-abb8-0aa49397069a\"},{\"content\":{\"connectorIds\":[\"Out1\",\"Out2\"],\"side\":\"RIGHT\"},\"type\":\"ConnectorPlacement.EquallySpacedRectSide\",\"uuid\":\"c7301fee-e42f-4254-87ba-788286fb640b\"},{\"content\":{\"connectorIds\":[\"In4\",\"In5\"],\"side\":\"TOP\"},\"type\":\"ConnectorPlacement.EquallySpacedRectSide\",\"uuid\":\"b96d884e-d525-4025-9411-9b9f9b32393f\"}]},\"type\":\"ConnectorPlacement.EquallySpacedConnector\",\"uuid\":\"b1e8dc5e-81c3-4a24-8e6d-921b13202a7f\"}],\"packageUris\":[\"http://schema.mathworks.com/mf0/Connector/R2020b\"],\"version\":\"1.0\"}"
  Logical Operator : Logic  Operator=NOT  AllPortsSameDT=off  OutDataTypeStr=boolean
  MO_ConsistantTau : Constant  Value=0
  MO_HealthLegdefault : Constant  Value=4.5
  MinimumTauGate : Subsystem
      settings: PortSchema="{\"entries\":[{\"content\":{\"sides\":[{\"content\":{\"connectorIds\":[\"In1\",\"In2\"]},\"type\":\"ConnectorPlacement.EquallySpacedRectSide\",\"uuid\":\"4d89c13b-f800-4481-b2e6-5754ccd4480d\"},{\"content\":{\"connectorIds\":[\"Out1\"],\"side\":\"RIGHT\"},\"type\":\"ConnectorPlacement.EquallySpacedRectSide\",\"uuid\":\"4c64cb92-33d7-49cd-aa82-02535cb98185\"},{\"content\":{\"side\":\"TOP\"},\"type\":\"ConnectorPlacement.EquallySpacedRectSide\",\"uuid\":\"dafdc7d9-c373-415f-80c5-51ad8948e064\"},{\"content\":{\"connectorIds\":[\"In3\"],\"side\":\"BOTTOM\"},\"type\":\"ConnectorPlacement.EquallySpacedRectSide\",\"uuid\":\"81b2cf25-e4b6-4f36-873c-2716d25d74ab\"}]},\"type\":\"ConnectorPlacement.EquallySpacedConnector\",\"uuid\":\"833ddaaa-290b-4880-823a-aa34ea5ccf1d\"}],\"packageUris\":[\"http://schema.mathworks.com/mf0/Connector/R2020b\"],\"version\":\"1.0\"}"
  SwingTauRelease : Subsystem
      settings: PortSchema="{\"entries\":[{\"content\":{\"sides\":[{\"content\":{\"connectorIds\":[\"In1\",\"In2\"]},\"type\":\"ConnectorPlacement.EquallySpacedRectSide\",\"uuid\":\"4d89c13b-f800-4481-b2e6-5754ccd4480d\"},{\"content\":{\"connectorIds\":[\"Out1\"],\"side\":\"RIGHT\"},\"type\":\"ConnectorPlacement.EquallySpacedRectSide\",\"uuid\":\"4c64cb92-33d7-49cd-aa82-02535cb98185\"},{\"content\":{\"connectorIds\":[\"In3\"],\"side\":\"TOP\"},\"type\":\"ConnectorPlacement.EquallySpacedRectSide\",\"uuid\":\"dafdc7d9-c373-415f-80c5-51ad8948e064\"},{\"content\":{\"side\":\"BOTTOM\"},\"type\":\"ConnectorPlacement.EquallySpacedRectSide\",\"uuid\":\"81b2cf25-e4b6-4f36-873c-2716d25d74ab\"}]},\"type\":\"ConnectorPlacement.EquallySpacedConnector\",\"uuid\":\"833ddaaa-290b-4880-823a-aa34ea5ccf1d\"}],\"packageUris\":[\"http://schema.mathworks.com/mf0/Connector/R2020b\"],\"version\":\"1.0\"}"
  Switch{,1..3} (4 alike) : Switch  Criteria=u2 > Threshold  SaturateOnIntegerOverflow=off  InputSameDT=off
  Right : Outport
  Left : Outport  Port=2
  wires:
  tau_e/1 -> MinimumTauGate/1(tau_e)
  Switch/1 -> LimitProtect/1(LeftHipMotorTorque)
  MO_HealthLegdefault/1 -> MinimumTauGate/2(In2), "?AllTimeDefault"/2, SwingTauRelease/2(In2)
  Switch1/1 -> LimitProtect/2(RightHipMotorTorque)
  LimitProtect/1(LeftHipMotorTorque_safe) -> Left/1
  LimitProtect/2(RightHipMotorTorque_safe) -> Right/1
  <LeftHipMotorActuralPosition>/1 -> LimitProtect/4(<LeftHipMotorActuralPosition>)
  <RightHipMotorActuralPosition>/1 -> LimitProtect/5(<RightHipMotorActuralPosition>)
  MinimumTauGate/1(Out1) -> Switch/3, Switch1/1
  LeftLowPass/1 -> ContactRelay/1
  FeetLoad/1 -> Demux/1, Demux1/1
  Demux/1 -> Switch2/1
  Demux/2 -> Switch2/3
  Logical Operator/1 -> Switch2/2
  Switch2/1 -> LeftLowPass/1
  ContactRelay/1 -> MinimumTauGate/3(In3)  "isAffectedStanding"
  WhichFoot/1 -> Switch1/2, LimitProtect/3(<WhichFoot>), Logical Operator/1, Switch/2, Switch3/2
  Demux1/1 -> Switch3/1
  Demux1/2 -> Switch3/3
  Switch3/1 -> LeftLowPass1/1
  LeftLowPass1/1 -> ContactRelay1/1
  ContactRelay1/1 -> SwingTauRelease/3(In3)  "isHealthyStanding"
  MO_ConsistantTau/1 -> SwingTauRelease/1(tau_e)
  "?AllTimeDefault"/1 -> Switch1/3, Switch/1
  SwingTauRelease/1(Out1) -> "?AllTimeDefault"/1

== system TestStructure/Robot/MotorPositonInit1 ==
  P : Inport
  BusOut : Inport  Port=2  OutDataTypeStr=Bus: SensingBusNew
  Enable : EnablePort
  Bus Creator : BusCreator  Inputs=4  OutDataTypeStr=Bus: ControlBusNew  NonVirtualBus=on
  Bus Selector : BusSelector  OutputSignals=LeftShoulderMotorActuralPosition,LeftShoulderMotorActuralVelocity
  Bus Selector1 : BusSelector  OutputSignals=RightShoulderMotorActuralPosition,RightShoulderMotorActuralVelocity
  Bus Selector2 : BusSelector  OutputSignals=LeftHipMotorActuralPosition,LeftHipMotorActuralVelocity
  Bus Selector3 : BusSelector  OutputSignals=RightHipMotorActuralPosition,RightHipMotorActuralVelocity
  Constant{,2..3,6} (4 alike) : Constant  Value=0
  Constant1 : Constant  OutDataTypeStr=double
  Constant4 : Constant  Value=0  OutDataTypeStr=double
  Constant5 : Constant
  Demux : Demux
  Discrete-Time Integrator : DiscreteIntegrator  SampleTime=-1  ICPrevOutput=DiscIntNeverNeededParam  ICPrevScaledInput=DiscIntNeverNeededParam
  Display5 : Display
  If Action Subsystem5 : Subsystem  TreatAsAtomicUnit=on
  If Action Subsystem6 : Subsystem  TreatAsAtomicUnit=on
  If2 : If  IfExpression=(u1 > 3.6)
  MATLAB Function1 : MATLAB Function  TreatAsAtomicUnit=on
  MATLAB Function2 : MATLAB Function  TreatAsAtomicUnit=on
  MATLAB Function3 : MATLAB Function  TreatAsAtomicUnit=on
  MATLAB Function4 : MATLAB Function  TreatAsAtomicUnit=on
  Merge1 : Merge
  Subsystem : Subsystem  Commented=on
  Subsystem1 : Subsystem
  Subsystem2 : Subsystem
  Subsystem3 : Subsystem
  Subsystem4 : Subsystem
  TaskFinished : Outport
  i_d : Outport  Port=2  OutDataTypeStr=Bus: ControlBusNew
  wires:
  Constant5/1 -> Discrete-Time Integrator/1
  If2/1 -> If Action Subsystem5/Action
  If2/2 -> If Action Subsystem6/Action
  If Action Subsystem6/1(Out1) -> Merge1/2
  Constant4/1 -> If Action Subsystem6/1(In1)
  Constant1/1 -> If Action Subsystem5/1(In1)
  If Action Subsystem5/1(Out1) -> Merge1/1
  Merge1/1 -> TaskFinished/1
  Bus Selector/2 -> Subsystem4/3(MotorVel)  "<LeftShoulderMotorActuralVelocity>"
  Bus Selector1/1 -> Subsystem1/2(MotorPos)  "<RightShoulderMotorActuralPosition>"
  Bus Selector1/2 -> Subsystem1/3(MotorVel)  "<RightShoulderMotorActuralVelocity>"
  MATLAB Function1/1(y) -> Subsystem1/1(MotorDesirePos)
  Constant/1 -> Bus Creator/1  "LeftShoulderMotorTorque"
  Subsystem3/1(MotorTorque) -> Bus Creator/4  "RightHipMotorTorque"
  Subsystem2/1(MotorTorque) -> Bus Creator/3  "LeftHipMotorTorque"
  Constant2/1 -> Bus Creator/2  "RightShoulderMotorTorque"
  Bus Creator/1 -> i_d/1
  BusOut/1 -> Bus Selector3/1, Bus Selector2/1, Bus Selector1/1, Bus Selector/1
  Bus Selector/1 -> Subsystem4/2(MotorPos)  "<LeftShoulderMotorActuralPosition>"
  Discrete-Time Integrator/1 -> MATLAB Function4/2(t), MATLAB Function3/2(t), MATLAB Function1/2(t), MATLAB Function2/2(t), If2/1, Display5/1
  Demux/1 -> MATLAB Function2/1(P)
  Demux/2 -> MATLAB Function1/1(P)
  MATLAB Function2/1(y) -> Subsystem4/1(MotorDesirePos)
  Demux/4 -> MATLAB Function4/1(P)
  Demux/3 -> MATLAB Function3/1(P)
  P/1 -> Demux/1
  Bus Selector2/1 -> Subsystem2/2(MotorPos)  "<LeftHipMotorActuralPosition>"
  Bus Selector2/2 -> Subsystem2/3(MotorVel)  "<LeftHipMotorActuralVelocity>"
  Bus Selector3/1 -> Subsystem3/2(MotorPos)  "<RightHipMotorActuralPosition>"
  Bus Selector3/2 -> Subsystem3/3(MotorVel)  "<RightHipMotorActuralVelocity>"
  MATLAB Function3/1(y) -> Subsystem2/1(MotorDesirePos)
  MATLAB Function4/1(y) -> Subsystem3/1(MotorDesirePos)

== system TestStructure/Bus/Subsystem/Enabled Subsystem ==
  In1 : Inport
  In2 : Inport  Port=2
  Enable : EnablePort
  Set Device State : slrealtimeethercatlib/Set SubDevice State  device_id=0  subdevice_name=Drive 3 (Elmo Drive )  sample_time=-1  subdevice_addr=1003  selected_subdevice=Term 1 (EK1100)  subdevice_found=1
  Out1 : Outport
  Out2 : Outport  Port=2
  wires:
  In1/1 -> Set Device State/1
  Set Device State/2 -> Out2/1
  In2/1 -> Set Device State/2
  Set Device State/1 -> Out1/1

== system TestStructure/Bus/Subsystem/Enabled Subsystem1 ==
  In3 : Inport
  Enable : EnablePort
  EtherCAT Async SDO Upload : slrealtimeethercatlib/EtherCAT Async SDO Upload  index=0x6075  subIndex=0  sig_type=uint32  sig_dim=1  device_id=0  subdevice_name=Drive 3 (Elmo Drive )  sample_time=-1  subdevice_addr=1003  selected_subdevice=Term 1 (EK1100)  timeout=3000  subdevice_found=1  complete=0
  Out3 : Outport
  Out4 : Outport  Port=2
  Out5 : Outport  Port=3
  wires:
  EtherCAT Async SDO Upload/3 -> Out5/1
  In3/1 -> EtherCAT Async SDO Upload/1
  EtherCAT Async SDO Upload/2 -> Out4/1
  EtherCAT Async SDO Upload/1 -> Out3/1

== system TestStructure/Bus/Subsystem/Enabled Subsystem2 ==
  In4 : Inport
  In5 : Inport  Port=2
  Enable : EnablePort
  EtherCAT Async SDO Download : slrealtimeethercatlib/EtherCAT Async SDO Download  index=0x6080  subIndex=0  sig_type=int32  sig_dim=1  device_id=0  subdevice_name=Drive 3 (Elmo Drive )  sample_time=-1  subdevice_addr=1003  selected_subdevice=Term 1 (EK1100)  timeout=3000  subdevice_found=1  complete=0
  Out6 : Outport
  Out7 : Outport  Port=2
  wires:
  EtherCAT Async SDO Download/2 -> Out7/1
  In4/1 -> EtherCAT Async SDO Download/1
  In5/1 -> EtherCAT Async SDO Download/2
  EtherCAT Async SDO Download/1 -> Out6/1

== system TestStructure/Bus/Subsystem/Enabled Subsystem3 ==
  In6 : Inport
  In7 : Inport  Port=2
  Enable : EnablePort
  EtherCAT Async SDO Download1 : slrealtimeethercatlib/EtherCAT Async SDO Download  index=0x6060  subIndex=0  sig_type=int8  sig_dim=1  device_id=0  subdevice_name=Drive 3 (Elmo Drive )  sample_time=-1  subdevice_addr=1003  selected_subdevice=Term 1 (EK1100)  timeout=2000  subdevice_found=1  complete=0
  Out8 : Outport
  Out9 : Outport  Port=2
  wires:
  In6/1 -> EtherCAT Async SDO Download1/1
  EtherCAT Async SDO Download1/1 -> Out8/1
  In7/1 -> EtherCAT Async SDO Download1/2
  EtherCAT Async SDO Download1/2 -> Out9/1

== system TestStructure/Bus/Subsystem/Enabled Subsystem4 ==
  In8 : Inport
  In9 : Inport  Port=2
  Enable : EnablePort
  Set Device State1 : slrealtimeethercatlib/Set SubDevice State  device_id=0  subdevice_name=Drive 3 (Elmo Drive )  sample_time=-1  subdevice_addr=1003  selected_subdevice=Term 1 (EK1100)  subdevice_found=1
  Out10 : Outport
  Out11 : Outport  Port=2
  wires:
  Set Device State1/1 -> Out10/1
  In8/1 -> Set Device State1/1
  In9/1 -> Set Device State1/2
  Set Device State1/2 -> Out11/1

== system TestStructure/Bus/Subsystem/Enabled Subsystem5 ==
  Enable : EnablePort
  Get Device State : slrealtimeethercatlib/Get SubDevice State  device_id=0  subdevice_name=Drive 3 (Elmo Drive )  sample_time=0.001  subdevice_addr=1003  selected_subdevice=Term 1 (EK1100)  timeout=500  subdevice_found=1
  Out12 : Outport
  wires:
  Get Device State/1 -> Out12/1

== system TestStructure/Bus/Subsystem/Enabled Subsystem6 ==
  In10 : Inport
  Enable : EnablePort
  EtherCAT PDO Receive1 : slrealtimeethercatlib/EtherCAT PDO Receive  Priority=2  sig_name=Drive 3 (Elmo Drive ).Inputs.Status word  sig_offset=1480  sig_type=uint16  type_size=16  sig_dim=1  device_id=0  sample_time=0.001000
  EtherCAT PDO Transmit1 : slrealtimeethercatlib/EtherCAT PDO Transmit  Priority=3  sig_name=Drive 3 (Elmo Drive ).Outputs.Control word  sig_offset=1448  sig_type=uint16  type_size=16  sig_dim=1  device_id=0  sample_time=0.001000
  Out13 : Outport
  wires:
  EtherCAT PDO Receive1/1 -> Out13/1
  In10/1 -> EtherCAT PDO Transmit1/1

== system TestStructure/Bus/Subsystem/Enabled Subsystem7 ==
  Enable : EnablePort
  EtherCAT PDO Receive2 : slrealtimeethercatlib/EtherCAT PDO Receive  Priority=2  sig_name=Drive 3 (Elmo Drive ).Inputs.Position actual value  sig_offset=1432  sig_type=int32  type_size=32  sig_dim=1  device_id=0  sample_time=0.001000
  Out1 : Outport
  wires:
  EtherCAT PDO Receive2/1 -> Out1/1

== system TestStructure/Bus/Subsystem4/Enabled Subsystem ==
  In1 : Inport
  In2 : Inport  Port=2
  Enable : EnablePort
  Set Device State : slrealtimeethercatlib/Set SubDevice State  device_id=0  subdevice_name=Drive 6 (Elmo Drive )  sample_time=-1  subdevice_addr=1006  selected_subdevice=Term 1 (EK1100)  subdevice_found=1
  Out1 : Outport
  Out2 : Outport  Port=2
  wires:
  In1/1 -> Set Device State/1
  Set Device State/2 -> Out2/1
  In2/1 -> Set Device State/2
  Set Device State/1 -> Out1/1

== system TestStructure/Bus/Subsystem4/Enabled Subsystem1 ==
  In3 : Inport
  Enable : EnablePort
  EtherCAT Async SDO Upload : slrealtimeethercatlib/EtherCAT Async SDO Upload  index=0x6075  subIndex=0  sig_type=uint32  sig_dim=1  device_id=0  subdevice_name=Drive 6 (Elmo Drive )  sample_time=-1  subdevice_addr=1006  selected_subdevice=Term 1 (EK1100)  timeout=3000  subdevice_found=1  complete=0
  Out3 : Outport
  Out4 : Outport  Port=2
  Out5 : Outport  Port=3
  wires:
  EtherCAT Async SDO Upload/3 -> Out5/1
  In3/1 -> EtherCAT Async SDO Upload/1
  EtherCAT Async SDO Upload/2 -> Out4/1
  EtherCAT Async SDO Upload/1 -> Out3/1

== system TestStructure/Bus/Subsystem4/Enabled Subsystem2 ==
  In4 : Inport
  In5 : Inport  Port=2
  Enable : EnablePort
  EtherCAT Async SDO Download : slrealtimeethercatlib/EtherCAT Async SDO Download  index=0x6080  subIndex=0  sig_type=int32  sig_dim=1  device_id=0  subdevice_name=Drive 6 (Elmo Drive )  sample_time=-1  subdevice_addr=1006  selected_subdevice=Term 1 (EK1100)  timeout=3000  subdevice_found=1  complete=0
  Out6 : Outport
  Out7 : Outport  Port=2
  wires:
  EtherCAT Async SDO Download/2 -> Out7/1
  In4/1 -> EtherCAT Async SDO Download/1
  In5/1 -> EtherCAT Async SDO Download/2
  EtherCAT Async SDO Download/1 -> Out6/1

== system TestStructure/Bus/Subsystem4/Enabled Subsystem3 ==
  In6 : Inport
  In7 : Inport  Port=2
  Enable : EnablePort
  EtherCAT Async SDO Download1 : slrealtimeethercatlib/EtherCAT Async SDO Download  index=0x6060  subIndex=0  sig_type=int8  sig_dim=1  device_id=0  subdevice_name=Drive 6 (Elmo Drive )  sample_time=-1  subdevice_addr=1006  selected_subdevice=Term 1 (EK1100)  timeout=2000  subdevice_found=1  complete=0
  Out8 : Outport
  Out9 : Outport  Port=2
  wires:
  In6/1 -> EtherCAT Async SDO Download1/1
  EtherCAT Async SDO Download1/1 -> Out8/1
  In7/1 -> EtherCAT Async SDO Download1/2
  EtherCAT Async SDO Download1/2 -> Out9/1

== system TestStructure/Bus/Subsystem4/Enabled Subsystem4 ==
  In8 : Inport
  In9 : Inport  Port=2
  Enable : EnablePort
  Set Device State1 : slrealtimeethercatlib/Set SubDevice State  device_id=0  subdevice_name=Drive 6 (Elmo Drive )  sample_time=-1  subdevice_addr=1006  selected_subdevice=Term 1 (EK1100)  subdevice_found=1
  Out10 : Outport
  Out11 : Outport  Port=2
  wires:
  Set Device State1/1 -> Out10/1
  In8/1 -> Set Device State1/1
  In9/1 -> Set Device State1/2
  Set Device State1/2 -> Out11/1

== system TestStructure/Bus/Subsystem4/Enabled Subsystem5 ==
  Enable : EnablePort
  Get Device State : slrealtimeethercatlib/Get SubDevice State  device_id=0  subdevice_name=Drive 6 (Elmo Drive )  sample_time=0.001  subdevice_addr=1006  selected_subdevice=Term 1 (EK1100)  timeout=500  subdevice_found=1
  Out12 : Outport
  wires:
  Get Device State/1 -> Out12/1

== system TestStructure/Bus/Subsystem4/Enabled Subsystem6 ==
  In10 : Inport
  Enable : EnablePort
  EtherCAT PDO Receive1 : slrealtimeethercatlib/EtherCAT PDO Receive  Priority=2  sig_name=Drive 6 (Elmo Drive ).Inputs.Status word  sig_offset=13280  sig_type=uint16  type_size=16  sig_dim=1  device_id=0  sample_time=0.001000
  EtherCAT PDO Transmit1 : slrealtimeethercatlib/EtherCAT PDO Transmit  Priority=3  sig_name=Drive 6 (Elmo Drive ).Outputs.Control word  sig_offset=13248  sig_type=uint16  type_size=16  sig_dim=1  device_id=0  sample_time=0.001000
  Out13 : Outport
  wires:
  EtherCAT PDO Receive1/1 -> Out13/1
  In10/1 -> EtherCAT PDO Transmit1/1

== system TestStructure/Bus/Subsystem4/Enabled Subsystem7 ==
  Enable : EnablePort
  EtherCAT PDO Receive2 : slrealtimeethercatlib/EtherCAT PDO Receive  Priority=2  sig_name=Drive 6 (Elmo Drive ).Inputs.Position actual value  sig_offset=13232  sig_type=int32  type_size=32  sig_dim=1  device_id=0  sample_time=0.001000
  Out1 : Outport
  wires:
  EtherCAT PDO Receive2/1 -> Out1/1
